simulink model "AMssb2"  (Simulink 8.3)
settings: Solver=ode45  StartTime=0.0  StopTime=1  RelTol=1e-3
undefined symbols (not defined in the file): get, hilbert
libraries: dspsnks4 x3, dspspect3 x3, dsparch4 x1
settings Model: Creator=maalmasr  LastModifiedBy=maalmasr
settings DataIOCC: SignalLoggingName=sigsOut
settings OptimizationCC: ExpressionDepthLimit=2147483647
settings DebuggingCC: SaveWithParameterizedLinksMsg=none  SignalResolutionControl=TryResolveAllWithWarning  SolverPrmCheckMsg=none  MultiTaskDSMMsg=warning  MultiTaskCondExecSysMsg=none  FcnCallInpInsideContextMsg=UseLocalSettings
settings HardwareCC: TargetUnknown=on
settings RTWCC: IncludeERTFirstTime=on

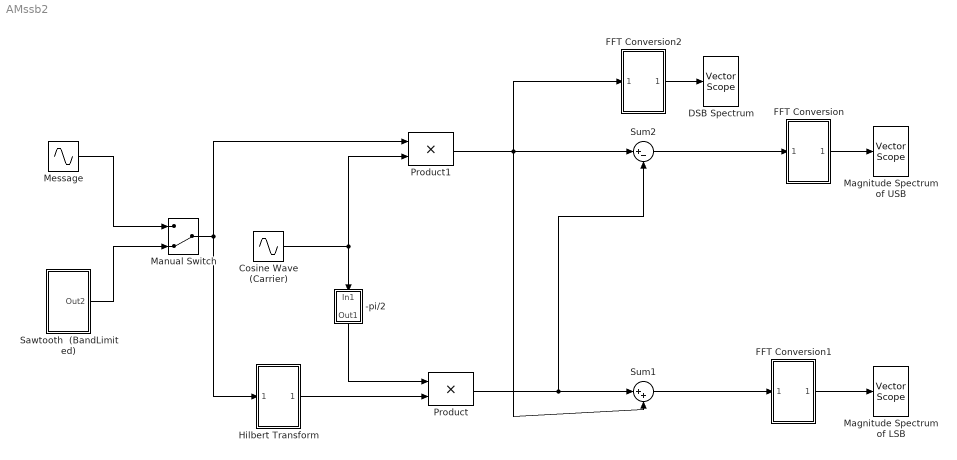
== system AMssb2 ==
  -pi/2 : Subsystem
  Cosine Wave (Carrier) : Sin  Frequency=2000*2*pi  Phase=pi/2  SampleTime=1/16000
      settings: AttributesFormatString=Frequency = %<Frequency>
  DSB Spectrum : dspsnks4/Vector Scope  ScopeProperties=off  Domain=Frequency  HorizSpan=1  DisplayProperties=off  AxisGrid=on  Memory=off  FrameNumber=on  AxisLegend=off  AxisZoom=off  OpenScopeAtSimStart=on  OpenScopeImmediately=off  FigPos=get(0,'defaultfigureposition')  AxisProperties=on  XUnits=Hertz  XRange=[0...Fs/2]  InheritXIncr=on  XIncr=1  XLabel=Time  XLimit=Auto  XMin=0  XMax=1  XStart=0  YUnits=Magnitude  YLabel=Amplitude  LineProperties=off  XAxisParamsVer=6.9
      settings: YMin=7.28583859910259e-018  YMax=0.262500000000009
  FFT Conversion : Subsystem
  FFT Conversion1 : Subsystem
  FFT Conversion2 : Subsystem
  Hilbert Transform : Subsystem
  Magnitude Spectrum of LSB : dspsnks4/Vector Scope  ScopeProperties=off  Domain=Frequency  HorizSpan=1  DisplayProperties=off  AxisGrid=on  Memory=off  FrameNumber=on  AxisLegend=off  AxisZoom=off  OpenScopeAtSimStart=on  OpenScopeImmediately=off  FigPos=get(0,'defaultfigureposition')  AxisProperties=on  XUnits=Hertz  XRange=[0...Fs/2]  InheritXIncr=on  XIncr=1  XLabel=Time  XLimit=Auto  XMin=0  XMax=1  XStart=0  YUnits=Magnitude  YLabel=Amplitude  LineProperties=off  XAxisParamsVer=6.9
      settings: YMin=6.07607110786267e-018  YMax=0.524999999999996
  "Magnitude Spectrum of USB " : dspsnks4/Vector Scope  ScopeProperties=off  Domain=Frequency  HorizSpan=1  DisplayProperties=off  AxisGrid=on  Memory=off  FrameNumber=on  AxisLegend=off  AxisZoom=off  OpenScopeAtSimStart=on  OpenScopeImmediately=off  FigPos=get(0,'defaultfigureposition')  AxisProperties=on  XUnits=Hertz  XRange=[0...Fs/2]  InheritXIncr=on  XIncr=1  XLabel=Time  XLimit=Auto  XMin=0  XMax=1  XStart=0  YUnits=Magnitude  YLabel=Amplitude  LineProperties=off  XAxisParamsVer=6.9
      settings: YMin=5.8703090278703e-018  YMax=0.524999999999996
  Manual Switch : ManualSwitch  CurrentSetting=0
  Message : Sin  Amplitude=0.8  Frequency=125*2*pi  SampleTime=1/16000
      settings: AttributesFormatString=Frequency = %<Frequency>\nm = %<Amplitude>
  Product : Product  SaturateOnIntegerOverflow=on  OutDataTypeStr=Inherit: Same as first input
  Product1 : Product  SaturateOnIntegerOverflow=on  OutDataTypeStr=Inherit: Same as first input
  Sawtooth  (BandLimited) : Subsystem
  Sum1 : Sum  Inputs=|++  SaturateOnIntegerOverflow=on
  Sum2 : Sum  Inputs=|+-  SaturateOnIntegerOverflow=on
  wires:
  Cosine Wave (Carrier)/1 -> Product1/2, -pi/2/1(In1)
  Product/1 -> Sum1/1, Sum2/2
  FFT Conversion/1(Out1) -> "Magnitude Spectrum of USB "/1
  Sum2/1 -> FFT Conversion/1(In1)
  FFT Conversion1/1(Out1) -> Magnitude Spectrum of LSB/1
  Sum1/1 -> FFT Conversion1/1(In1)
  Product1/1 -> Sum1/2, FFT Conversion2/1(In1), Sum2/1
  Hilbert Transform/1(Out1) -> Product/2
  -pi/2/1(Out1) -> Product/1
  FFT Conversion2/1(Out1) -> DSB Spectrum/1
  Manual Switch/1 -> Hilbert Transform/1(In1), Product1/1
  Message/1 -> Manual Switch/1
  Sawtooth  (BandLimited)/1(Out2) -> Manual Switch/2

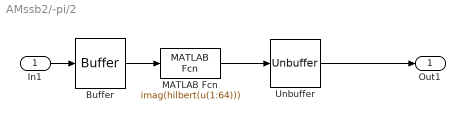
== system AMssb2/-pi/2 ==
  In1 : Inport
  Buffer : Buffer  TreatMby1Signals=One channel
  MATLAB Fcn : MATLABFcn  MATLABFcn=imag(hilbert(u(1:64)))  Output1D=off
  Unbuffer : Unbuffer  SampleBasedProcessing=Same as frame based
  Out1 : Outport
  wires:
  MATLAB Fcn/1 -> Unbuffer/1
  In1/1 -> Buffer/1
  Unbuffer/1 -> Out1/1
  Buffer/1 -> MATLAB Fcn/1

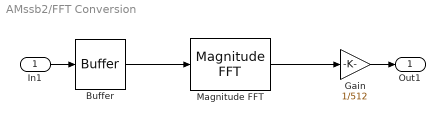
== system AMssb2/FFT Conversion ==
  In1 : Inport
  Buffer : Buffer  N=512  TreatMby1Signals=One channel
  Gain : Gain  Gain=1/512  SaturateOnIntegerOverflow=on  OutDataTypeStr=Inherit: Same as input  ParamDataTypeStr=Inherit: Same as input
  Magnitude FFT : dspspect3/Magnitude FFT  mag_or_magsq=Magnitude  FFTImplementation=Auto  fftLenInherit=on  fftsize=256  WrapInput=on
  Out1 : Outport
  wires:
  Buffer/1 -> Magnitude FFT/1
  Magnitude FFT/1 -> Gain/1
  In1/1 -> Buffer/1
  Gain/1 -> Out1/1

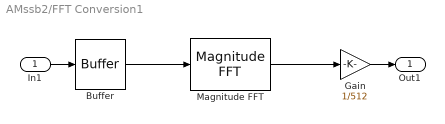
== system AMssb2/FFT Conversion1 ==
  In1 : Inport
  Buffer : Buffer  N=512  TreatMby1Signals=One channel
  Gain : Gain  Gain=1/512  SaturateOnIntegerOverflow=on  OutDataTypeStr=Inherit: Same as input  ParamDataTypeStr=Inherit: Same as input
  Magnitude FFT : dspspect3/Magnitude FFT  mag_or_magsq=Magnitude  FFTImplementation=Auto  fftLenInherit=on  fftsize=256  WrapInput=on
  Out1 : Outport
  wires:
  Buffer/1 -> Magnitude FFT/1
  Magnitude FFT/1 -> Gain/1
  In1/1 -> Buffer/1
  Gain/1 -> Out1/1

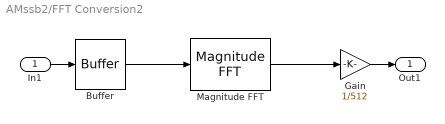
== system AMssb2/FFT Conversion2 ==
  In1 : Inport
  Buffer : Buffer  N=512  TreatMby1Signals=One channel
  Gain : Gain  Gain=1/512  SaturateOnIntegerOverflow=on  OutDataTypeStr=Inherit: Same as input  ParamDataTypeStr=Inherit: Same as input
  Magnitude FFT : dspspect3/Magnitude FFT  mag_or_magsq=Magnitude  FFTImplementation=Auto  fftLenInherit=on  fftsize=256  WrapInput=on
  Out1 : Outport
  wires:
  Buffer/1 -> Magnitude FFT/1
  Magnitude FFT/1 -> Gain/1
  In1/1 -> Buffer/1
  Gain/1 -> Out1/1

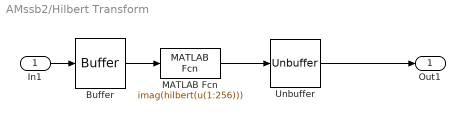
== system AMssb2/Hilbert Transform ==
  In1 : Inport
  Buffer : Buffer  N=256  TreatMby1Signals=One channel
  MATLAB Fcn : MATLABFcn  MATLABFcn=imag(hilbert(u(1:256)))  Output1D=off
  Unbuffer : Unbuffer  SampleBasedProcessing=Same as frame based
  Out1 : Outport
  wires:
  MATLAB Fcn/1 -> Unbuffer/1
  In1/1 -> Buffer/1
  Unbuffer/1 -> Out1/1
  Buffer/1 -> MATLAB Fcn/1

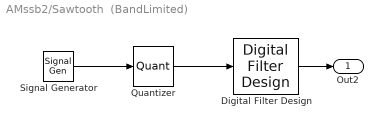
== system AMssb2/Sawtooth  (BandLimited) ==
  Digital Filter Design : dsparch4/Digital Filter Design  mwdsp_browser_bugfix_var=off
  Quantizer : Quantizer  QuantizationInterval=0.05  SampleTime=1/16000
  Signal Generator : SignalGenerator  WaveForm=sawtooth  Frequency=125
  Out2 : Outport
  wires:
  Signal Generator/1 -> Quantizer/1
  Digital Filter Design/1 -> Out2/1
  Quantizer/1 -> Digital Filter Design/1
